simulink model "MATLABxuexi06"  (R2016a)
settings: Solver=VariableStepAuto  StartTime=0.0  StopTime=0.1  RelTol=1e-3
libraries: powerlib x13, powerlib_meascontrol x3, dspstat3 x1
settings Model: Creator=24535  LastModifiedBy=24535

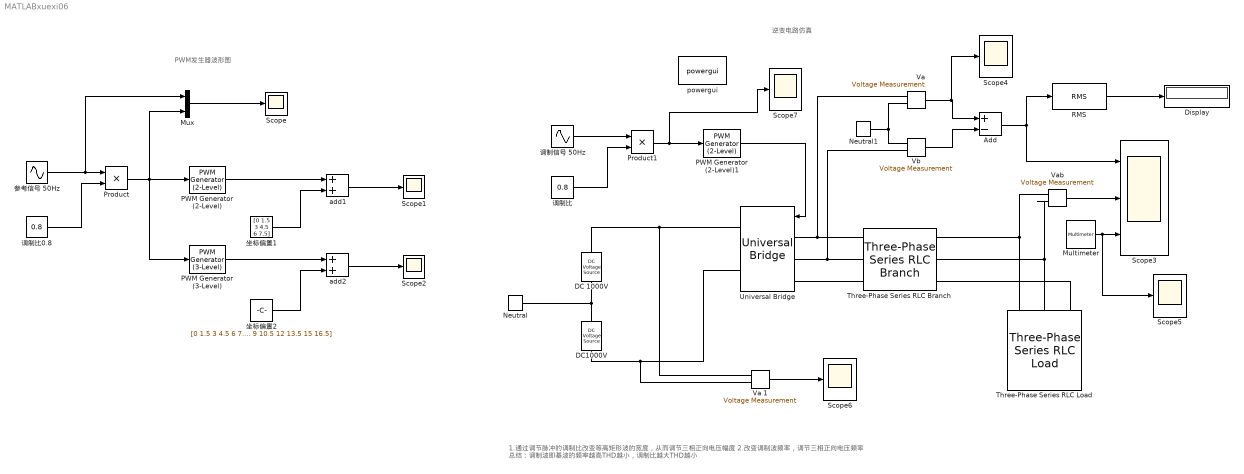
== system MATLABxuexi06 ==
  note: 1.通过调节脉冲的调制比改变等高矩形波的宽度，从而调节三相正向电压幅度
      |
      | 2.改变调制波频率，调节三相正向电压频率
      |
      | 总结：调制波即基波的频率越高THD越小，调制比越大THD越小
  note: 逆变电路仿真
  note: PWM发生器波形图
  Add : Sum  Inputs=+-
  DC 1000V : powerlib/Electrical Sources/DC Voltage Source  Amplitude=1000  Measurements=None
  DC1000V : powerlib/Electrical Sources/DC Voltage Source  Amplitude=1000  Measurements=None
  Display : Display
      settings: Decimation=100
  Multimeter : powerlib/Measurements/Multimeter  PhasorSimulation=off  OutputType=Complex  sel=14  L=22  Gain=1  yselected={'Iag: Three-Phase Series RLC Load'};  PSBOutputType=1  PSBequivalent=0  AxesSetting=[0,0.1,-100,100]  Display=0  SavedBlockNames=-11
  Mux : Mux  Inputs=2
  Neutral : powerlib/Elements/Neutral  LConnTagsString=a  NodeNumber=1
  Neutral1 : powerlib/Elements/Neutral  LConnTagsString=a  NodeNumber=1
  PWM Generator (2-Level) : powerlib_meascontrol/Pulse & Signal Generators/PWM Generator (2-Level)  ModulatorType=Three-phase bridge (6 pulses)  ModulatorMode=Unsynchronized  Fc=33*50  Pc=90  nF=27  MinMax="[ -1  1 ]"  SamplingTechnique=Natural  ModulatingSignals=off  m=0.8  Freq=60  Phase=0  Ts=0  ShowCarrierOutport=off
  PWM Generator (2-Level)1 : powerlib_meascontrol/Pulse & Signal Generators/PWM Generator (2-Level)  ModulatorType=Three-phase bridge (6 pulses)  ModulatorMode=Unsynchronized  Fc=33*50  Pc=90  nF=27  MinMax="[ -1  1 ]"  SamplingTechnique=Natural  ModulatingSignals=off  m=0.8  Freq=60  Phase=0  Ts=0  ShowCarrierOutport=off
  PWM Generator (3-Level) : powerlib_meascontrol/Pulse & Signal Generators/PWM Generator (3-Level)  ModulatorType=Three-phase bridge (12 pulses)  ModulatorMode=Unsynchronized  nF=27  Fc=33*50  ModulatingSignals=off  m=0.8  Freq=60  Phase=0  Ts=0
  Product : Product
  Product1 : Product
  RMS : dspstat3/RMS  run=off  reset_popup=None  InputProcessing=Columns as channels (frame based)  directionMode=Each column  dimension=1
  Scope{,1..2,4..7} (7 alike) : Scope
  Scope3 : Scope  NumInputPorts=3
  Three-Phase Series RLC Branch : powerlib/Elements/Three-Phase Series RLC Branch  LConnTagsString=A|B|C  RConnTagsString=A|B|C  BranchType=RL  Resistance=10e-3  Inductance=100e-6  Capacitance=1e-6  Measurements=None
  Three-Phase Series RLC Load : powerlib/Elements/Three-Phase Series RLC Load  LConnTagsString=A|B|C  Configuration=Y (grounded)  NominalVoltage=2000  Vabc=[1e3 1e3 1e3]  Vabcp=[1e3 1e3 1e3]  NominalFrequency=50  UnbalancedPower=off  ActivePower=500e3  InductivePower=100e3  CapacitivePower=0  Pabc=[10e3 9e3 11e3]  QLabc=[100 90 110]  QCabc=[100 90 110]  Pabcp=[10e3 9e3 11e3]  QLabcp=[100 90 110]  QCabcp=[100 90 110]  Measurements=Branch voltages and currents  LoadType=constant Z
  Universal Bridge : powerlib/Power Electronics/Universal Bridge  Arms=3  SnubberResistance=10  SnubberCapacitance=0.47e-6  Device=IGBT / Diodes  Ron=1e-4  Lon=0  ForwardVoltages="[  0.7  0.7  ]"  ForwardVoltage=0  GTOparameters=[ 10e-6 , 20e-6 ]  IGBTparameters=[ 1e-6 , 2e-6 ]  Measurements=All voltages and currents  Measurements_2=None  converterType=Rectifier
  "Va " : powerlib/Measurements/Voltage Measurement  PhasorSimulation=off  OutputType=Complex  PSBequivalent=0
  Va 1 : powerlib/Measurements/Voltage Measurement  PhasorSimulation=off  OutputType=Complex  PSBequivalent=0
  "Vab " : powerlib/Measurements/Voltage Measurement  PhasorSimulation=off  OutputType=Complex  PSBequivalent=0
  "Vb " : powerlib/Measurements/Voltage Measurement  PhasorSimulation=off  OutputType=Complex  PSBequivalent=0
  add1 : Sum
  add2 : Sum
  powergui : powerlib/powergui  Priority=1  SimulationMode=Discrete  SolverType=Tustin/Backward Euler (TBE)  SampleTime=2e-6  frequency=60  SPID=off  DisableSnubberDevices=off  DisableRonSwitches=off  DisableVfSwitches=off  SwTol=0  DisplayEquations=off  Interpol=off  ExternalGateDelay=off  methode=off  Ts=10  FunctionMessages=off  echomessages=off  HookPort=off  EnableUseOfTLC=off  x0status=blocks  frequencyindice=0  Pbase=100e6  ErrMax=1e-4  Iterations=50  UnitsV=kV  UnitsW=MW  buscounter=0  RestoreLinks=warning  ResistiveCurrentMeasurement=off  Frange=[0:2:500]  Ylog=off  Xlog=on  ShowGrid=off  save=off  variable=ZData  structure=ScopeData5  ZoomFFT=off  StartTime=0.0  cycles=4  DisplayStyle=1  fundamental=50  FreqAxis=off  MaxFrequency=6000  frequencyindicesteady=1  RmsSteady=1  display=off
  参考信号 50Hz : Sin  Frequency=100*pi  Phase=[0 -2*pi/3 2*pi/3]  SampleTime=0
  坐标偏置1 : Constant  Value=[0 1.5 3 4.5 6 7.5]
  坐标偏置2 : Constant  Value=[0 1.5 3 4.5 6 7.5 9 10.5 12 13.5 15 16.5]
  调制信号 50Hz : Sin  Frequency=100*pi  Phase=[0 -2*pi/3 2*pi/3]  SampleTime=0
  调制比 : Constant  Value=0.8
  调制比0.8 : Constant  Value=0.8
  wires:
  参考信号 50Hz/1 -> Mux/1, Product/1
  调制比0.8/1 -> Product/2
  Product/1 -> PWM Generator (3-Level)/1, Mux/2, PWM Generator (2-Level)/1
  PWM Generator (2-Level)/1 -> add1/1
  Mux/1 -> Scope/1
  add1/1 -> Scope1/1
  PWM Generator (3-Level)/1 -> add2/1
  add2/1 -> Scope2/1
  坐标偏置1/1 -> add1/2
  坐标偏置2/1 -> add2/2
  调制信号 50Hz/1 -> Product1/1
  调制比/1 -> Product1/2
  Product1/1 -> Scope7/1, PWM Generator (2-Level)1/1
  PWM Generator (2-Level)1/1 -> Universal Bridge/1
  Multimeter/1 -> Scope5/1, Scope3/3
  "Vab "/1 -> Scope3/2
  RMS/1 -> Display/1
  "Va "/1 -> Scope4/1, Add/1
  "Vb "/1 -> Add/2
  Add/1 -> Scope3/1, RMS/1
  Va 1/1 -> Scope6/1
  connections:
  DC1000V/RConn1 -- Neutral/LConn1 -- DC 1000V/LConn1
  DC 1000V/RConn1 -- Va 1/LConn1 -- Universal Bridge/RConn1
  Universal Bridge/RConn2 -- Va 1/LConn2 -- DC1000V/LConn1
  Three-Phase Series RLC Branch/LConn1 -- "Va "/LConn1 -- Universal Bridge/LConn1
  Universal Bridge/LConn2 -- "Vb "/LConn1 -- Three-Phase Series RLC Branch/LConn2
  Three-Phase Series RLC Branch/LConn3 -- Universal Bridge/LConn3
  Three-Phase Series RLC Load/LConn1 -- Three-Phase Series RLC Branch/RConn1 -- "Vab "/LConn1
  Three-Phase Series RLC Branch/RConn2 -- Three-Phase Series RLC Load/LConn2 -- "Vab "/LConn2
  Three-Phase Series RLC Branch/RConn3 -- Three-Phase Series RLC Load/LConn3
  Neutral1/LConn1 -- "Vb "/LConn2 -- "Va "/LConn2
